simulink model "nmpc_block_2014a"  (R2014a)
settings: Solver=ode45  StartTime=0.0  StopTime=tfin  FixedStep=1  RelTol=1e-3
values from neighbouring files (symbols this model uses):
  K = nmpc_design(par)    [main_HCW.m]    (also in nmpc_design_template.m)
undefined symbols (not defined in the file or in its folder): nmpc_law
settings Model: CovSFcnEnable=on  Creator=carlonovara  LastModifiedBy=carlonovara
settings DataIOCC: LimitDataPoints=off  SaveFormat=StructureWithTime
settings DebuggingCC: MergeDetectMultiDrivingBlocksExec=error  SolverPrmCheckMsg=none  FrameProcessingCompatibilityMsg=error
settings HardwareCC: ProdBitPerPointer=64  ProdLargestAtomicFloat=Float  ProdIntDivRoundTo=Zero  ProdEndianess=LittleEndian  ProdHWDeviceType=Specified
settings ModelReferenceCC: PropagateSignalLabelsOutOfModel=on

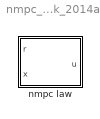
== system nmpc_block_2014a ==
  nmpc law : Subsystem

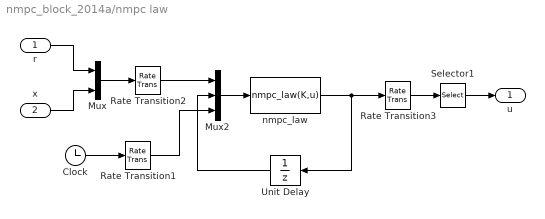
== system nmpc_block_2014a/nmpc law ==
  r : Inport
  x : Inport  Port=2
  Clock : Clock
  Mux : Mux  Inputs=2
  Mux2 : Mux  Inputs=3
  Rate Transition1 : RateTransition  OutPortSampleTime=K.Ts
  Rate Transition2 : RateTransition  OutPortSampleTime=K.Ts
  Rate Transition3 : RateTransition  OutPortSampleTime=0
  Selector1 : Selector  InputPortWidth=K.nc  IndexOptions=Index vector (dialog)  Indices=1:K.nu  OutputSizes=1
  Unit Delay : UnitDelay  InitialCondition=zeros(K.nc,1)  SampleTime=K.Ts  HasFrameUpgradeWarning=on
  nmpc_law : MATLABFcn  MATLABFcn=nmpc_law(K,u)  OutputDimensions=K.nc
  u : Outport
  wires:
  Rate Transition3/1 -> Selector1/1
  Unit Delay/1 -> Mux2/2
  Mux2/1 -> nmpc_law/1
  Rate Transition2/1 -> Mux2/1
  nmpc_law/1 -> Rate Transition3/1, Unit Delay/1
  Mux/1 -> Rate Transition2/1
  r/1 -> Mux/1
  x/1 -> Mux/2
  Selector1/1 -> u/1
  Rate Transition1/1 -> Mux2/3
  Clock/1 -> Rate Transition1/1
